simulink model "quad_control_fala_2015"  (Simulink 8.7)
settings: Solver=ode3  StartTime=0.0  StopTime=20  FixedStep=0.01  RelTol=1e-3
InitFcn:
  | % --- Inner loop gains --------
  | %Kp_roll = 0.05;
  | %Kp_pitch = 0.05;
  | %Kp_yaw = 0.2;
  | 
  | %Ki_roll = 0.01;
  | %Ki_pitch = 0.01;
  | %Ki_yaw = 0.1;
  | 
  | %Kd_roll = 0.004;
  | %Kd_pitch = 0.004;
  | %Kd_yaw = 0.04;
  | 
  | %D_roll = 0.04;
  | %D_pitch = 0.04;
  | %D_yaw = 0.2;
  | % --------------------------
  | 
  | % --- Outer loop gains --------
  | Kp_altitude = 8;
  | Kp_pos_x = 10;
  | Kp_pos_y = 10;
  | 
  | Ki_altitude = 0.1;
  | Ki_pos_x = 5;
  | Ki_pos_y = 5;
  | 
  | Kd_altitude = 5;
  | Kd_pos_x = 5;
  | Kd_pos_y = 5;
  | % --------------------------
  | 
  | % --- Saturation limits --------
  | pos_upper_limit = 1;
  | pos_lower_limit = -1;
  | 
  | mvel_upper_limit = 10;
  | mvel_lower_limit = 0;
  | % --------------------------
  | 
  | global clientID;
  | clientID=-1;
values from neighbouring files (symbols this model uses):
  D_pitch = Pitch_controller_coef_escolhidos(3)    [FALA_LA_Inner_Controllers.m]
  D_roll = Roll_controller_coef_escolhidos(3)    [FALA_LA_Inner_Controllers.m]
  D_yaw = Yaw_controller_coef_escolhidos(3)    [FALA_LA_Inner_Controllers.m]
  Kp_pitch = Pitch_controller_coef_escolhidos(1)    [FALA_LA_Inner_Controllers.m]
  Kp_roll = Roll_controller_coef_escolhidos(1)    [FALA_LA_Inner_Controllers.m]
  Kp_yaw = Yaw_controller_coef_escolhidos(1)    [FALA_LA_Inner_Controllers.m]
undefined symbols (not defined in the file or in its folder): Angular, Linear
libraries: simulink_extras x6, robotlib x4, aerolibtransform2 x2
settings Model: Creator=kleber  LastModifiedBy=kleber
settings DebuggingCC: UnderspecifiedInitializationDetection=Simplified  MergeDetectMultiDrivingBlocksExec=error  SolverPrmCheckMsg=warning
settings ConfigComp: CovSFcnEnable=off

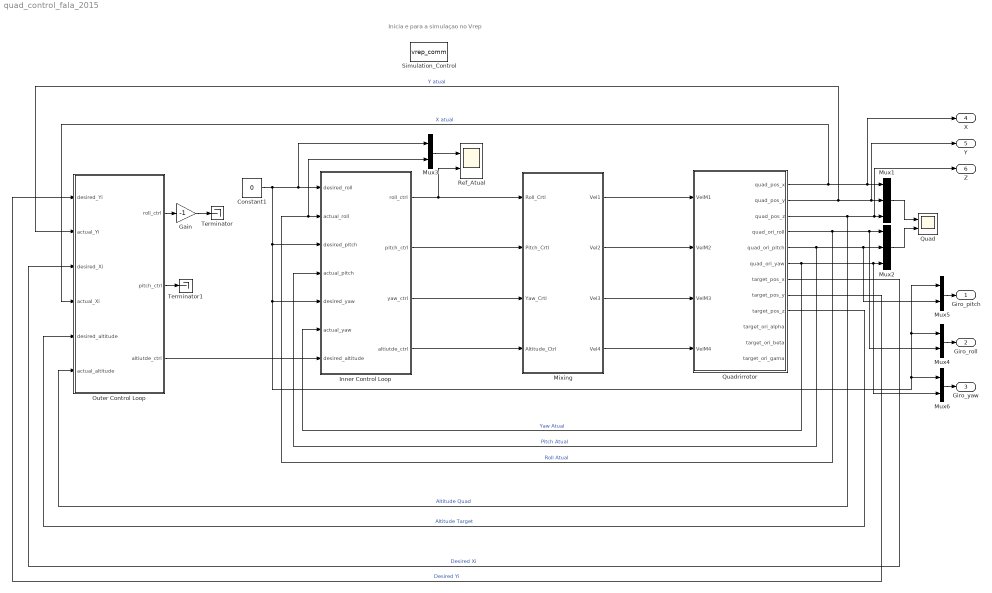
== system quad_control_fala_2015 ==
  note: Inicia e para a simulaçao no Vrep
  Constant1 : Constant  Value=0
  Gain : Gain  Gain=-1
  Inner Control Loop : Subsystem
  Mixing : Subsystem
  Mux1 : Mux  Inputs=3
  Mux2 : Mux  Inputs=3
  Mux{3..6} (4 alike) : Mux  Inputs=2
  Outer Control Loop : Subsystem
  Quad : Scope  NumInputPorts=2
  Quadrirrotor : Subsystem
  Ref_Atual : Scope  NumInputPorts=2
  Simulation_Control : S-Function  FunctionName=vrep_comm  SFunctionDeploymentMode=off  EnableBusSupport=off
  Terminator : Terminator
  Terminator1 : Terminator
  Giro_pitch : Outport
  Giro_roll : Outport  Port=2
  Giro_yaw : Outport  Port=3
  X : Outport  Port=4
  Y : Outport  Port=5
  Z : Outport  Port=6
  wires:
  Mux1/1 -> Quad/1
  Mux2/1 -> Quad/2
  Quadrirrotor/5(quad_ori_pitch) -> Mux5/2, Mux2/2, Inner Control Loop/4(actual_pitch)  "Pitch Atual"
  Quadrirrotor/4(quad_ori_roll) -> Mux4/2, Mux2/1, Mux3/2, Inner Control Loop/2(actual_roll)  "Roll Atual"
  Quadrirrotor/1(quad_pos_x) -> Outer Control Loop/4(actual_Xi), X/1, Mux1/1  "X atual"
  Quadrirrotor/3(quad_pos_z) -> Z/1, Mux1/3, Outer Control Loop/6(actual_altitude)  "Altitude Quad"
  Quadrirrotor/6(quad_ori_yaw) -> Mux6/2, Mux2/3, Inner Control Loop/6(actual_yaw)  "Yaw Atual"
  Mixing/1(Vel1) -> Quadrirrotor/1(VelM1)
  Mixing/2(Vel2) -> Quadrirrotor/2(VelM2)
  Mixing/3(Vel3) -> Quadrirrotor/3(VelM3)
  Mixing/4(Vel4) -> Quadrirrotor/4(VelM4)
  Inner Control Loop/3(yaw_ctrl) -> Mixing/3(Yaw_Crtl)
  Inner Control Loop/1(roll_ctrl) -> Ref_Atual/2, Mixing/1(Roll_Crtl)
  Inner Control Loop/4(altiutde_ctrl) -> Mixing/4(Altitude_Ctrl)
  Inner Control Loop/2(pitch_ctrl) -> Mixing/2(Pitch_Crtl)
  Outer Control Loop/3(altiutde_ctrl) -> Inner Control Loop/7(desired_altitude)
  Quadrirrotor/2(quad_pos_y) -> Outer Control Loop/2(actual_Yi), Y/1, Mux1/2  "Y atual"
  Quadrirrotor/7(target_pos_x) -> Outer Control Loop/3(desired_Xi)  "Desired Xi"
  Quadrirrotor/8(target_pos_y) -> Outer Control Loop/1(desired_Yi)  "Desired Yi"
  Quadrirrotor/9(target_pos_z) -> Outer Control Loop/5(desired_altitude)  "Altitude Target"
  Constant1/1 -> Mux6/1, Mux4/1, Mux5/1, Inner Control Loop/5(desired_yaw), Inner Control Loop/3(desired_pitch), Inner Control Loop/1(desired_roll), Mux3/1
  Mux3/1 -> Ref_Atual/1
  Outer Control Loop/1(roll_ctrl) -> Gain/1
  Gain/1 -> Terminator/1
  Outer Control Loop/2(pitch_ctrl) -> Terminator1/1
  Mux4/1 -> Giro_roll/1
  Mux5/1 -> Giro_pitch/1
  Mux6/1 -> Giro_yaw/1

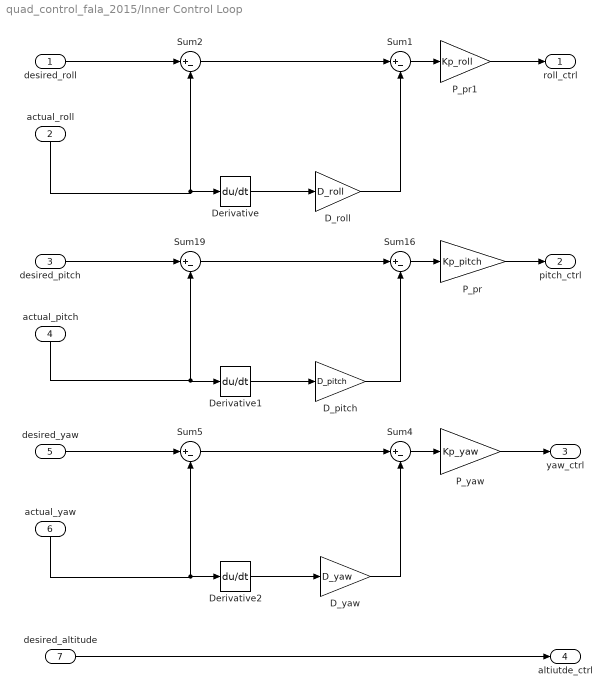
== system quad_control_fala_2015/Inner Control Loop ==
  desired_roll : Inport
  actual_roll : Inport  Port=2
  desired_pitch : Inport  Port=3
  actual_pitch : Inport  Port=4
  desired_yaw : Inport  Port=5
  actual_yaw : Inport  Port=6
  desired_altitude : Inport  Port=7
  D_pitch : Gain  Gain=D_pitch
  D_roll : Gain  Gain=D_roll
  D_yaw : Gain  Gain=D_yaw
  Derivative : Derivative
  Derivative1 : Derivative
  Derivative2 : Derivative
  P_pr : Gain  Gain=Kp_pitch
  P_pr1 : Gain  Gain=Kp_roll
  P_yaw : Gain  Gain=Kp_yaw
  Sum{1..2,4..5,16,19} (6 alike) : Sum  Inputs=|+-
  roll_ctrl : Outport
  pitch_ctrl : Outport  Port=2
  yaw_ctrl : Outport  Port=3
  altiutde_ctrl : Outport  Port=4
  wires:
  desired_altitude/1 -> altiutde_ctrl/1
  Sum19/1 -> Sum16/1
  Sum16/1 -> P_pr/1
  P_pr/1 -> pitch_ctrl/1
  D_pitch/1 -> Sum16/2
  Derivative1/1 -> D_pitch/1
  actual_pitch/1 -> Sum19/2, Derivative1/1
  Sum2/1 -> Sum1/1
  Sum1/1 -> P_pr1/1
  D_roll/1 -> Sum1/2
  Derivative/1 -> D_roll/1
  desired_pitch/1 -> Sum19/1
  actual_roll/1 -> Sum2/2, Derivative/1
  desired_roll/1 -> Sum2/1
  actual_yaw/1 -> Sum5/2, Derivative2/1
  Sum4/1 -> P_yaw/1
  Derivative2/1 -> D_yaw/1
  D_yaw/1 -> Sum4/2
  Sum5/1 -> Sum4/1
  desired_yaw/1 -> Sum5/1
  P_pr1/1 -> roll_ctrl/1
  P_yaw/1 -> yaw_ctrl/1

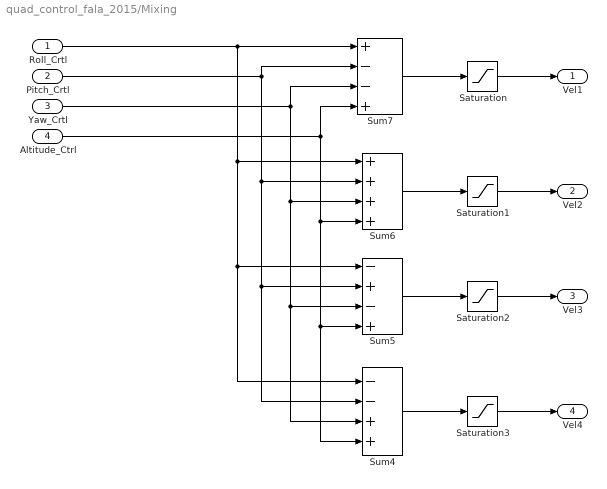
== system quad_control_fala_2015/Mixing ==
  Roll_Crtl : Inport
  Pitch_Crtl : Inport  Port=2
  Yaw_Crtl : Inport  Port=3
  Altitude_Ctrl : Inport  Port=4
  Saturation{,1..3} (4 alike) : Saturate  UpperLimit=mvel_upper_limit  LowerLimit=mvel_lower_limit
  Sum4 : Sum  Inputs=--++
  Sum5 : Sum  Inputs=-+-+
  Sum6 : Sum  Inputs=++++
  Sum7 : Sum  Inputs=+--+
  Vel1 : Outport
  Vel2 : Outport  Port=2
  Vel3 : Outport  Port=3
  Vel4 : Outport  Port=4
  wires:
  Yaw_Crtl/1 -> Sum4/3, Sum5/3, Sum6/3, Sum7/3
  Roll_Crtl/1 -> Sum4/1, Sum5/1, Sum6/1, Sum7/1
  Pitch_Crtl/1 -> Sum4/2, Sum5/2, Sum6/2, Sum7/2
  Altitude_Ctrl/1 -> Sum4/4, Sum5/4, Sum6/4, Sum7/4
  Sum7/1 -> Saturation/1
  Saturation/1 -> Vel1/1
  Sum6/1 -> Saturation1/1
  Saturation1/1 -> Vel2/1
  Sum5/1 -> Saturation2/1
  Saturation2/1 -> Vel3/1
  Sum4/1 -> Saturation3/1
  Saturation3/1 -> Vel4/1

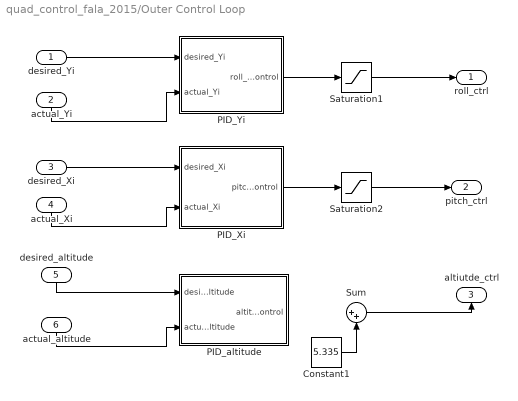
== system quad_control_fala_2015/Outer Control Loop ==
  desired_Yi : Inport
  actual_Yi : Inport  Port=2
  desired_Xi : Inport  Port=3
  actual_Xi : Inport  Port=4
  desired_altitude : Inport  Port=5
  actual_altitude : Inport  Port=6
  Constant1 : Constant  Value=5.335
  PID_Xi : Subsystem
  PID_Yi : Subsystem
  PID_altitude : Subsystem
  Saturation1 : Saturate  UpperLimit=pos_upper_limit  LowerLimit=pos_lower_limit
  Saturation2 : Saturate  UpperLimit=pos_upper_limit  LowerLimit=pos_lower_limit
  Sum : Sum  Inputs=|++
  roll_ctrl : Outport
  pitch_ctrl : Outport  Port=2
  altiutde_ctrl : Outport  Port=3
  wires:
  PID_Yi/1(roll_control) -> Saturation1/1
  PID_Xi/1(pitch_control) -> Saturation2/1
  desired_Yi/1 -> PID_Yi/1(desired_Yi)
  Sum/1 -> altiutde_ctrl/1
  desired_Xi/1 -> PID_Xi/1(desired_Xi)
  actual_Xi/1 -> PID_Xi/2(actual_Xi)
  desired_altitude/1 -> PID_altitude/1(desired_altitude)
  actual_altitude/1 -> PID_altitude/2(actual_altitude)
  actual_Yi/1 -> PID_Yi/2(actual_Yi)
  Saturation1/1 -> roll_ctrl/1
  Saturation2/1 -> pitch_ctrl/1
  Constant1/1 -> Sum/2

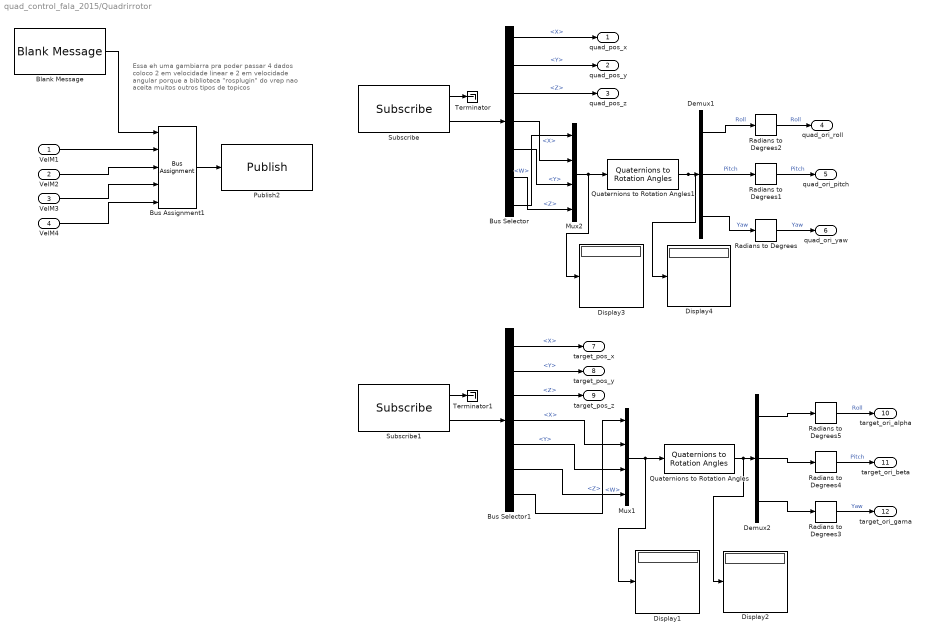
== system quad_control_fala_2015/Quadrirrotor ==
  note: Essa eh uma gambiarra pra poder passar 4 dados coloco 2 em velocidade linear e 2 em velocidade angular porque a biblioteca "rosplugin" do vrep nao aceita muitos outros tipos de topicos
  VelM1 : Inport
  VelM2 : Inport  Port=2
  VelM3 : Inport  Port=3
  VelM4 : Inport  Port=4
  Blank Message : robotlib/Blank Message  SourceLibraryInfo=This block requires Robotics System Toolbox  messageType=geometry_msgs/Twist  SampleTime=inf
  Bus Assignment1 : BusAssignment  DialogController=Simulink.DDGSource_BusAssignment  AssignedSignals=Linear.X,Linear.Y,Angular.X,Angular.Y
  Bus Selector : BusSelector  OutputSignals=Pose.Position.X,Pose.Position.Y,Pose.Position.Z,Pose.Orientation.X,Pose.Orientation.Y,Pose.Orientation.Z,Pose.Orientation.W
  Bus Selector1 : BusSelector  OutputSignals=Pose.Position.X,Pose.Position.Y,Pose.Position.Z,Pose.Orientation.X,Pose.Orientation.Y,Pose.Orientation.Z,Pose.Orientation.W
  Demux1 : Demux  Outputs=3
  Demux2 : Demux  Outputs=3
  Display{1..4} (4 alike) : Display
  Mux1 : Mux
  Mux2 : Mux
  Publish2 : robotlib/Publish  SourceLibraryInfo=This block requires Robotics System Toolbox  topicSource=Select from ROS network  topic=/control_signals  messageType=geometry_msgs/Twist  messageQueueLength=105
  Quaternions to Rotation Angles : aerolibtransform2/Quaternions to Rotation Angles  rotationOrder=XYZ
  Quaternions to Rotation Angles1 : aerolibtransform2/Quaternions to Rotation Angles  rotationOrder=XYZ
  Radians to Degrees{,1..5} (6 alike) : simulink_extras/Transformations/Radians to Degrees
  Subscribe : robotlib/Subscribe  SourceLibraryInfo=This block requires Robotics System Toolbox  topicSource=Select from ROS network  topic=/quad_pos_ang  messageType=geometry_msgs/PoseStamped  sampleTime=-1  messageQueueLength=51
  Subscribe1 : robotlib/Subscribe  SourceLibraryInfo=This block requires Robotics System Toolbox  topicSource=Select from ROS network  topic=/target_pos_ang  messageType=geometry_msgs/PoseStamped  sampleTime=-1  messageQueueLength=51
  Terminator : Terminator
  Terminator1 : Terminator
  quad_pos_x : Outport
  quad_pos_y : Outport  Port=2
  quad_pos_z : Outport  Port=3
  quad_ori_roll : Outport  Port=4
  quad_ori_pitch : Outport  Port=5
  quad_ori_yaw : Outport  Port=6
  target_pos_x : Outport  Port=7
  target_pos_y : Outport  Port=8
  target_pos_z : Outport  Port=9
  target_ori_alpha : Outport  Port=10
  target_ori_beta : Outport  Port=11
  target_ori_gama : Outport  Port=12
  wires:
  VelM1/1 -> Bus Assignment1/2
  Bus Selector/1 -> quad_pos_x/1  "<X>"
  Bus Selector/2 -> quad_pos_y/1  "<Y>"
  Bus Selector/3 -> quad_pos_z/1  "<Z>"
  Radians to Degrees2/1 -> quad_ori_roll/1  "Roll"
  Radians to Degrees1/1 -> quad_ori_pitch/1  "Pitch"
  Radians to Degrees/1 -> quad_ori_yaw/1  "Yaw"
  Bus Selector1/1 -> target_pos_x/1  "<X>"
  Bus Selector1/3 -> target_pos_z/1  "<Z>"
  Demux2/1 -> Radians to Degrees5/1
  Demux2/2 -> Radians to Degrees4/1
  Demux2/3 -> Radians to Degrees3/1
  Demux1/3 -> Radians to Degrees/1  "Yaw"
  Demux1/2 -> Radians to Degrees1/1  "Pitch"
  Demux1/1 -> Radians to Degrees2/1  "Roll"
  Radians to Degrees5/1 -> target_ori_alpha/1  "Roll"
  Radians to Degrees4/1 -> target_ori_beta/1  "Pitch"
  Radians to Degrees3/1 -> target_ori_gama/1  "Yaw"
  Bus Assignment1/1 -> Publish2/1
  Blank Message/1 -> Bus Assignment1/1
  Mux1/1 -> Display1/1, Quaternions to Rotation Angles/1
  Bus Selector1/5 -> Mux1/3  "<Y>"
  Bus Selector1/6 -> Mux1/4  "<Z>"
  Bus Selector1/7 -> Mux1/1  "<W>"
  Quaternions to Rotation Angles/1 -> Display2/1, Demux2/1
  Subscribe/2 -> Bus Selector/1
  Subscribe1/2 -> Bus Selector1/1
  Bus Selector1/2 -> target_pos_y/1  "<Y>"
  Subscribe/1 -> Terminator/1
  Subscribe1/1 -> Terminator1/1
  Bus Selector1/4 -> Mux1/2  "<X>"
  Mux2/1 -> Quaternions to Rotation Angles1/1, Display3/1
  Bus Selector/5 -> Mux2/3  "<Y>"
  Bus Selector/6 -> Mux2/4  "<Z>"
  Bus Selector/7 -> Mux2/1  "<W>"
  Quaternions to Rotation Angles1/1 -> Demux1/1, Display4/1
  Bus Selector/4 -> Mux2/2  "<X>"
  VelM2/1 -> Bus Assignment1/3
  VelM3/1 -> Bus Assignment1/4
  VelM4/1 -> Bus Assignment1/5

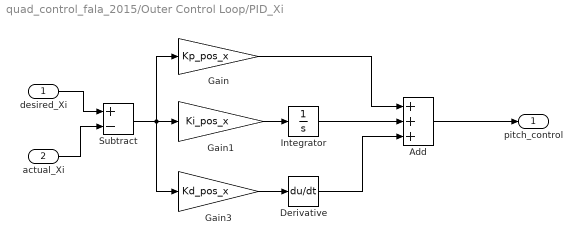
== system quad_control_fala_2015/Outer Control Loop/PID_Xi ==
  desired_Xi : Inport
  actual_Xi : Inport  Port=2
  Add : Sum  Inputs=+++
  Derivative : Derivative
  Gain : Gain  Gain=Kp_pos_x
  Gain1 : Gain  Gain=Ki_pos_x
  Gain3 : Gain  Gain=Kd_pos_x
  Integrator : Integrator
  Subtract : Sum  Inputs=+-
  pitch_control : Outport
  wires:
  Gain3/1 -> Derivative/1
  Gain1/1 -> Integrator/1
  Gain/1 -> Add/1
  Add/1 -> pitch_control/1
  desired_Xi/1 -> Subtract/1
  Subtract/1 -> Gain/1, Gain1/1, Gain3/1
  actual_Xi/1 -> Subtract/2
  Integrator/1 -> Add/2
  Derivative/1 -> Add/3

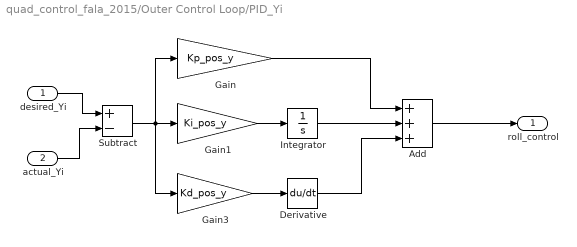
== system quad_control_fala_2015/Outer Control Loop/PID_Yi ==
  desired_Yi : Inport
  actual_Yi : Inport  Port=2
  Add : Sum  Inputs=+++
  Derivative : Derivative
  Gain : Gain  Gain=Kp_pos_y
  Gain1 : Gain  Gain=Ki_pos_y
  Gain3 : Gain  Gain=Kd_pos_y
  Integrator : Integrator
  Subtract : Sum  Inputs=+-
  roll_control : Outport
  wires:
  Gain3/1 -> Derivative/1
  Gain1/1 -> Integrator/1
  Subtract/1 -> Gain3/1, Gain1/1, Gain/1
  desired_Yi/1 -> Subtract/1
  Add/1 -> roll_control/1
  Gain/1 -> Add/1
  actual_Yi/1 -> Subtract/2
  Integrator/1 -> Add/2
  Derivative/1 -> Add/3

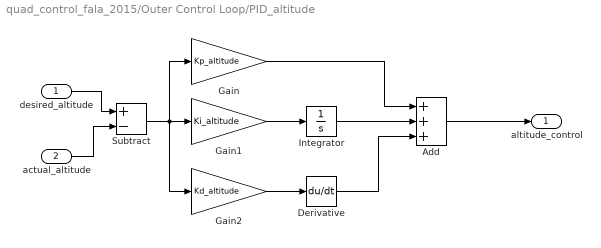
== system quad_control_fala_2015/Outer Control Loop/PID_altitude ==
  desired_altitude : Inport
  actual_altitude : Inport  Port=2
  Add : Sum  Inputs=+++
  Derivative : Derivative
  Gain : Gain  Gain=Kp_altitude
  Gain1 : Gain  Gain=Ki_altitude
  Gain2 : Gain  Gain=Kd_altitude
  Integrator : Integrator
  Subtract : Sum  Inputs=+-
  altitude_control : Outport
  wires:
  Gain2/1 -> Derivative/1
  Gain1/1 -> Integrator/1
  Gain/1 -> Add/1
  Add/1 -> altitude_control/1
  actual_altitude/1 -> Subtract/2
  desired_altitude/1 -> Subtract/1
  Subtract/1 -> Gain/1, Gain1/1, Gain2/1
  Integrator/1 -> Add/2
  Derivative/1 -> Add/3
